simulink model "OutputVoltage_J"  (R2020b)
settings: Solver=VariableStepAuto  StartTime=0.0  StopTime=t_final  RelTol=1e-3
values from neighbouring files (symbols this model uses):
  SOC_initial = 0.5    [Run_Model.m]
  x2_initial = 0    [Run_Model.m]
settings Model: Creator=moonjihoon  LastModifiedBy=moonjihoon

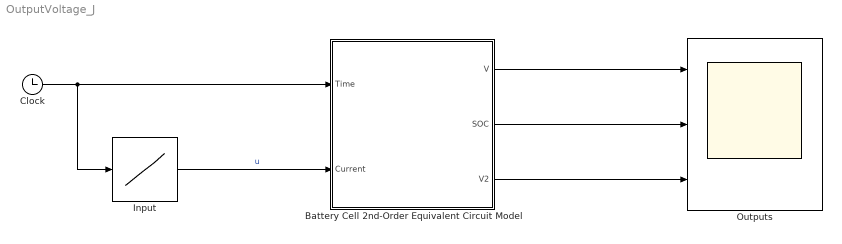
== system OutputVoltage_J ==
  Battery Cell 2nd-Order Equivalent Circuit Model : Subsystem
  Clock : Clock
  Input : Lookup_n-D  NumberOfTableDimensions=1  BreakpointsForDimension1=t  Table=u  InternalRulePriority=Speed  RndMeth=Simplest  InputSameDT=on
  Outputs : Scope  NumInputPorts=3
  wires:
  Clock/1 -> Input/1, Battery Cell 2nd-Order Equivalent Circuit Model/1(Time)
  Input/1 -> Battery Cell 2nd-Order Equivalent Circuit Model/2(Current)  "u"
  Battery Cell 2nd-Order Equivalent Circuit Model/1(V) -> Outputs/1
  Battery Cell 2nd-Order Equivalent Circuit Model/2(SOC) -> Outputs/2
  Battery Cell 2nd-Order Equivalent Circuit Model/3(V2) -> Outputs/3

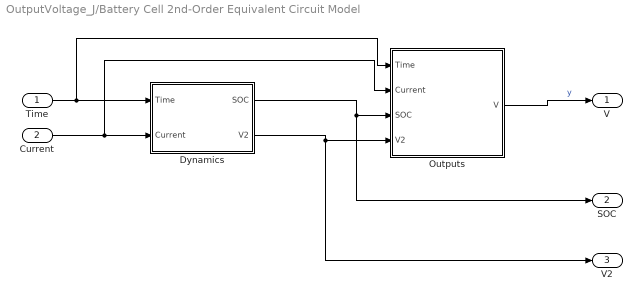
== system OutputVoltage_J/Battery Cell 2nd-Order Equivalent Circuit Model ==
  Time : Inport
  Current : Inport  Port=2
  Dynamics : Subsystem
  Outputs : Subsystem
  V : Outport
  SOC : Outport  Port=2
  V2 : Outport  Port=3
  wires:
  Dynamics/1(SOC) -> SOC/1, Outputs/3(SOC)
  Dynamics/2(V2) -> V2/1, Outputs/4(V2)
  Current/1 -> Outputs/2(Current), Dynamics/2(Current)
  Outputs/1(V) -> V/1  "y"
  Time/1 -> Outputs/1(Time), Dynamics/1(Time)

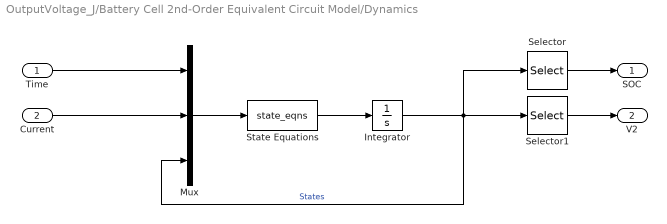
== system OutputVoltage_J/Battery Cell 2nd-Order Equivalent Circuit Model/Dynamics ==
  Time : Inport
  Current : Inport  Port=2
  Integrator : Integrator  InitialCondition=[SOC_initial;x2_initial]
  Mux : Mux  Inputs=3
  Selector : Selector  InputPortWidth=2  IndexOptions=Index vector (dialog)  Indices=[1]  OutputSizes=1
  Selector1 : Selector  InputPortWidth=2  IndexOptions=Index vector (dialog)  Indices=[2]  OutputSizes=1
  State Equations : MATLABFcn  MATLABFcn=state_eqns
  SOC : Outport
  V2 : Outport  Port=2
  wires:
  Current/1 -> Mux/2
  Integrator/1 -> Mux/3, Selector/1, Selector1/1  "States"
  Mux/1 -> State Equations/1
  Selector1/1 -> V2/1
  Selector/1 -> SOC/1
  Time/1 -> Mux/1
  State Equations/1 -> Integrator/1

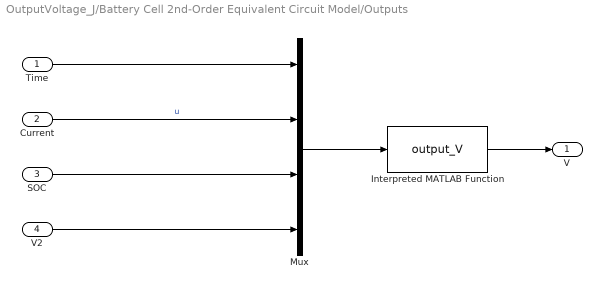
== system OutputVoltage_J/Battery Cell 2nd-Order Equivalent Circuit Model/Outputs ==
  Time : Inport
  Current : Inport  Port=2
  SOC : Inport  Port=3
  V2 : Inport  Port=4
  Interpreted MATLAB Function : MATLABFcn  MATLABFcn=output_V
  Mux : Mux
  V : Outport
  wires:
  Current/1 -> Mux/2  "u"
  SOC/1 -> Mux/3
  V2/1 -> Mux/4
  Mux/1 -> Interpreted MATLAB Function/1
  Interpreted MATLAB Function/1 -> V/1
  Time/1 -> Mux/1
